simulink model "free_fall (1)"  (R2017b)
settings: Solver=VariableStepAuto  StartTime=0.0  StopTime=10.0  RelTol=1e-3
undefined symbols (not defined in the file): magnitude
settings Model: Creator=Siddharth  LastModifiedBy=Siddharth

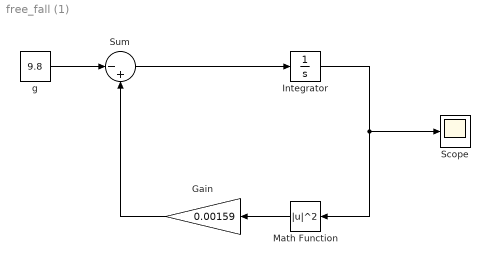
== system free_fall (1) ==
  Gain : Gain  Gain=0.00159
  Integrator : Integrator
  Math Function : Math  Operator=magnitude^2  SaturateOnIntegerOverflow=on
  Scope : Scope
  Sum : Sum  Inputs=|-+
  g : Constant  Value=9.8
  wires:
  g/1 -> Sum/1
  Sum/1 -> Integrator/1
  Gain/1 -> Sum/2
  Math Function/1 -> Gain/1
  Integrator/1 -> Scope/1, Math Function/1
